simulink model "to_F411RE"  (R2021b)
settings: Solver=VariableStepAuto  StartTime=0.0  StopTime=inf  RelTol=1e-3
libraries: instrumentseriallib x3
settings Model: Creator=imark  LastModifiedBy=imark

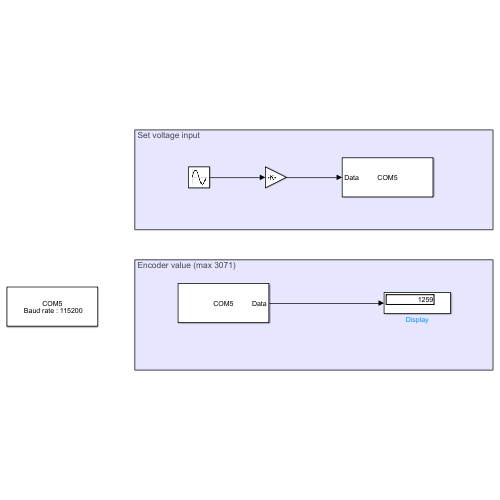
[thumbnail: Simulink's stored preview of the top-level diagram]
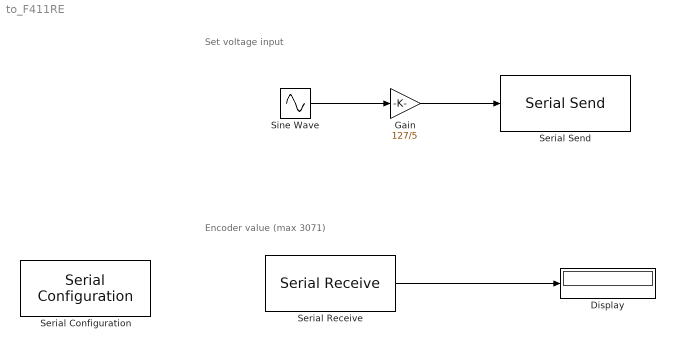
== system to_F411RE ==
  note: Encoder value (max 3071)
  note: Set voltage input
  Display : Display
  Gain : Gain  Gain=127/5  OutDataTypeStr=int8
  Serial Configuration : instrumentseriallib/Serial Configuration  Priority=-200000  Port=COM5  ComPort=COM5  BaudRate=115200  DataBits=8  Parity=none  StopBits=1  ByteOrder=little-endian  FlowControl=none  Timeout=10  SimulateUsing=Interpreted execution  BlockInModel=on
  Serial Receive : instrumentseriallib/Serial Receive  Priority=1  Port=COM5  ComPort=COM5  DataType=uint16  SaveDataType=uint8  ToggleHeader=on  Header=[73 109 64 99]  ToggleTerminator=on  Terminator=Custom terminator  CustomTerminator=[126]  ToggleDataSize=on  DataSize=[1 1]  EnableBlockingMode=on  ActionDataUnavailable=Output last received value  ActionWhenDataUnavailable=Output last received value  CustomValue=0  SampleTime=-1  SimulateUsing=Interpreted execution  BlockInModel=on
  Serial Send : instrumentseriallib/Serial Send  Priority=1  Port=COM5  ComPort=COM5  Header=[73 109 64 99]  Terminator=Custom terminator  CustomTerminator=[126]  EnableBlockingMode=on  SimulateUsing=Interpreted execution  BlockInModel=on
  Sine Wave : Sin  Amplitude=5  Frequency=1/20
  wires:
  Serial Receive/1 -> Display/1
  Sine Wave/1 -> Gain/1
  Gain/1 -> Serial Send/1
